simulink model "hjuloppheng_sim"  (R2024a)
settings: Solver=VariableStepAuto  StartTime=0.0  StopTime=10.0  RelTol=1e-3
values from neighbouring files (symbols this model uses):
  B = 500    [hjuloppheng.m]
  K1 = 20000    [hjuloppheng.m]
  K2 = 10000    [hjuloppheng.m]
  M1 = 40    [hjuloppheng.m]
  M2 = 250    [hjuloppheng.m]
settings Model: Creator=rune  LastModifiedBy=rune

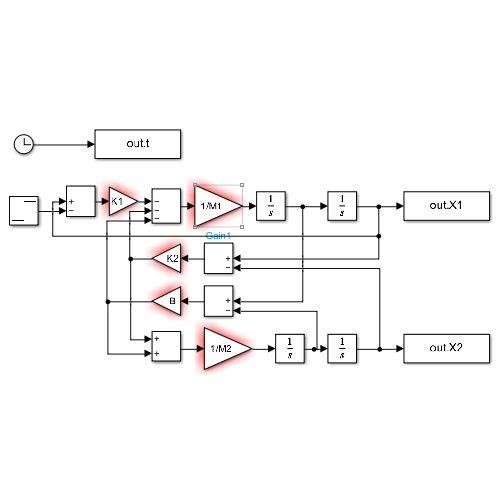
[thumbnail: Simulink's stored preview of the top-level diagram]
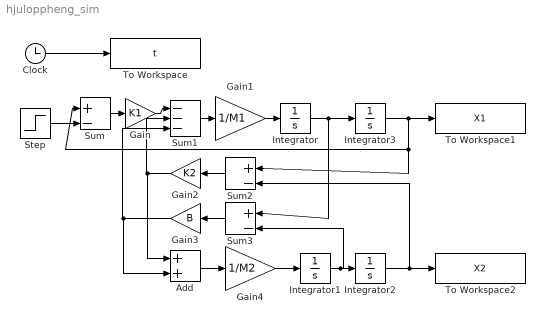
== system hjuloppheng_sim ==
  Add : Sum
  Clock : Clock
  Gain : Gain  Gain=K1
  Gain1 : Gain  Gain=1/M1
  Gain2 : Gain  Gain=K2
  Gain3 : Gain  Gain=B
  Gain4 : Gain  Gain=1/M2
  Integrator{,1..3} (4 alike) : Integrator
  Step : Step  SampleTime=0
  Sum : Sum  Inputs=|+-
  Sum1 : Sum  Inputs=|---
  Sum2 : Sum  Inputs=|+-
  Sum3 : Sum  Inputs=|+-
  To Workspace : ToWorkspace  VariableName=t  SampleTime=-1
  To Workspace1 : ToWorkspace  VariableName=X1  SampleTime=-1
  To Workspace2 : ToWorkspace  VariableName=X2  SampleTime=-1
  wires:
  Clock/1 -> To Workspace/1
  Step/1 -> Sum/2
  Sum/1 -> Gain/1
  Gain/1 -> Sum1/1
  Sum1/1 -> Gain1/1
  Gain1/1 -> Integrator/1
  Gain2/1 -> Add/1, Sum1/2
  Gain3/1 -> Add/2, Sum1/3
  Sum2/1 -> Gain2/1
  Sum3/1 -> Gain3/1
  Add/1 -> Gain4/1
  Gain4/1 -> Integrator1/1
  Integrator1/1 -> Sum3/2, Integrator2/1
  Integrator2/1 -> To Workspace2/1, Sum2/2
  Integrator/1 -> Sum3/1, Integrator3/1
  Integrator3/1 -> Sum2/1, Sum/1, To Workspace1/1
